simulink model "expert_random"  (R2023a)
settings: Solver=VariableStepAuto  StartTime=0.0  StopTime=1000  RelTol=1e-3
values from neighbouring files (symbols this model uses):
  A1 = 0.0154    [expert_pid_script.m]    (also in optimizer.m; parametros.m; variables.mat)
  A2 = 5e-5    (= 5e-05)    [expert_pid_script.m]    (also in optimizer.m; parametros.m; variables.mat)
  az = 1    [expert_pid_script.m]    (also in optimizer.m; parametros.m = 0.5; variables.mat = 0.5)
  g = 9.8    [expert_pid_script.m]    (also in optimizer.m; parametros.m; variables.mat)
  Q_star = ro*A2*az*sqrt(2*g*H_star)    [expert_pid_script.m]    (also in optimizer.m; parametros.m; variables.mat = 0.0616238590158)
  ro = 1000    [expert_pid_script.m]    (also in optimizer.m; parametros.m; variables.mat)
  semilla = 751    [parametros.m]    (also in variables.mat)
  st = 0.001    [parametros.m]    (also in variables.mat)
undefined symbols (not defined in the file or in its folder): DiscIntNeverNeededParam
settings Model: Creator=empg0  LastModifiedBy=empg0
settings DebuggingCC: AlgebraicLoopMsg=none

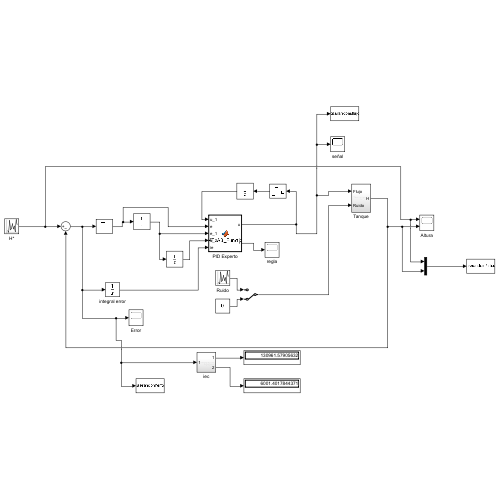
[thumbnail: Simulink's stored preview of the top-level diagram]
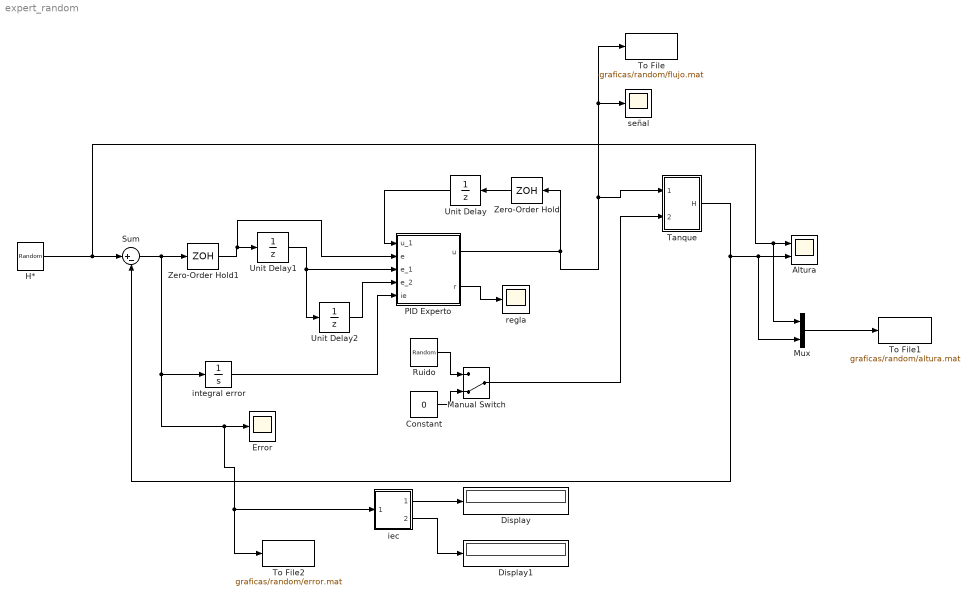
== system expert_random ==
  Altura : Scope  NumInputPorts=2
  Constant : Constant  Value=0
  Display : Display
  Display1 : Display
  Error : Scope
  H* : UniformRandomNumber  Minimum=0  Maximum=0.62  Seed=semilla  SampleTime=200
  Manual Switch : ManualSwitch  CurrentSetting=0
  Mux : Mux  Inputs=2
  PID Experto : MATLAB Function  TreatAsAtomicUnit=on
  Ruido : UniformRandomNumber  Minimum=-Q_star*0.3  Maximum=Q_star*0.3  Seed=140  SampleTime=0.5
  Sum : Sum  Inputs=|+-
  Tanque : Subsystem
  To File : ToFile  Filename=graficas/random/flujo.mat  MatrixName=flujo  SampleTime=0.25
  To File1 : ToFile  Filename=graficas/random/altura.mat  MatrixName=altura  SampleTime=0.25
  To File2 : ToFile  Filename=graficas/random/error.mat  MatrixName=error  SampleTime=0.25
  Unit Delay : UnitDelay  SampleTime=st  HasFrameUpgradeWarning=on
  Unit Delay1 : UnitDelay  SampleTime=st  HasFrameUpgradeWarning=on
  Unit Delay2 : UnitDelay  SampleTime=st  HasFrameUpgradeWarning=on
  Zero-Order Hold : ZeroOrderHold  SampleTime=st
  Zero-Order Hold1 : ZeroOrderHold  SampleTime=st
  iec : Subsystem
  integral error : Integrator
  regla : Scope
  señal : Scope
  wires:
  Tanque/1(H) -> Sum/2, Mux/2, Altura/2
  Manual Switch/1 -> Tanque/2(Ruido)
  H*/1 -> Mux/1, Altura/1, Sum/1
  Ruido/1 -> Manual Switch/1
  Constant/1 -> Manual Switch/2
  Sum/1 -> Zero-Order Hold1/1, To File2/1, iec/1(In1), Error/1, integral error/1
  Zero-Order Hold1/1 -> Unit Delay1/1, PID Experto/2(e)
  Unit Delay2/1 -> PID Experto/4(e_2)
  Unit Delay1/1 -> Unit Delay2/1, PID Experto/3(e_1)
  integral error/1 -> PID Experto/5(ie)
  PID Experto/1(u) -> To File/1, señal/1, Tanque/1(Flujo), Zero-Order Hold/1
  Zero-Order Hold/1 -> Unit Delay/1
  Unit Delay/1 -> PID Experto/1(u_1)
  PID Experto/2(r) -> regla/1
  iec/1(Out1) -> Display/1
  Mux/1 -> To File1/1
  iec/2(Out2) -> Display1/1

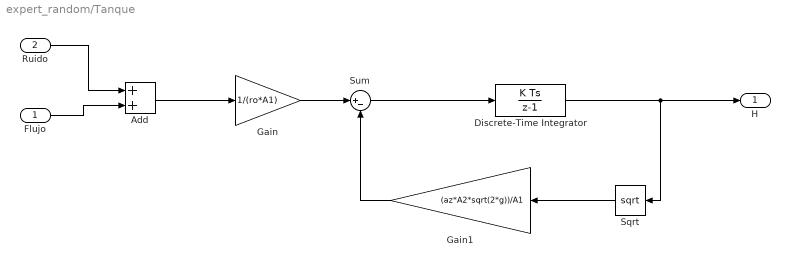
== system expert_random/Tanque ==
  Flujo : Inport
  Ruido : Inport  Port=2
  Add : Sum
  Discrete-Time Integrator : DiscreteIntegrator  SampleTime=st  LimitOutput=on  UpperSaturationLimit=0.62  LowerSaturationLimit=0  ICPrevOutput=DiscIntNeverNeededParam  ICPrevScaledInput=DiscIntNeverNeededParam
  Gain : Gain  Gain=1/(ro*A1)
  Gain1 : Gain  Gain=(az*A2*sqrt(2*g))/A1
  Sqrt : Sqrt
  Sum : Sum  Inputs=|+-
  H : Outport
  wires:
  Gain/1 -> Sum/1
  Sqrt/1 -> Gain1/1
  Gain1/1 -> Sum/2
  Add/1 -> Gain/1
  Flujo/1 -> Add/2
  Ruido/1 -> Add/1
  Sum/1 -> Discrete-Time Integrator/1
  Discrete-Time Integrator/1 -> H/1, Sqrt/1

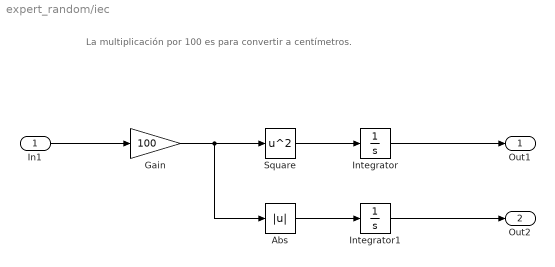
== system expert_random/iec ==
  note: La multiplicación por 100 es para convertir a centímetros.
  In1 : Inport
  Abs : Abs  SaturateOnIntegerOverflow=off
  Gain : Gain  Gain=100
  Integrator : Integrator
  Integrator1 : Integrator
  Square : Math  Operator=square  SignedPower=on  RndMeth=Zero
  Out1 : Outport
  Out2 : Outport  Port=2
  wires:
  Square/1 -> Integrator/1
  Integrator/1 -> Out1/1
  In1/1 -> Gain/1
  Gain/1 -> Abs/1, Square/1
  Integrator1/1 -> Out2/1
  Abs/1 -> Integrator1/1

== matlab function expert_random/PID Experto ==
  data: u_1 input; e input; u output; e_1 input; e_2 input; ie input; r output
function [u, r] = MATLAB_Function(u_1, e, e_1, e_2, ie)
    
    %st = load("sampling_time.mat");
    % Constantes
    H_max = 0.62;
    M1 = H_max/2;
    M2 = H_max/4;
    epsilon = 0.001; % cambié de 0.01 a 0.005
    st = 0.001; % 0.1 -> 0.001

    Qmax = 0.1; % flujo máximo
    Qmin = 0; % flujo mínimo
    
    k1 = 4.9321;
    k2 = 0.033265;
    kp = 1.06160;
    ki = 0.05; %0.03014;
    kd = -2.20023;

    de = e - e_1;
    de_1 = e_1 - e_2;
    if abs(e) > M1 % regla 1
        r = 1;
        if e > 0
            u = Qmax;
        else
            u = Qmin;
        end
    elseif abs(e) <= epsilon % regla 5
        r = 5;
        u = u_1 + kp*(e - e_1) + ki*ie;
    elseif e*de < 0 && de*de_1 < 0 % regla 4
        r = 4;
        if abs(e) >= M2
            u = u_1 + k1*kp*e;
        else
            u = u_1 + k2*kp*e;
        end
    elseif (e*de < 0 && de*de_1 > 0) || e == 0 % regla 3
        r = 3;
        u = u_1;
    elseif e*de > 0 || de == 0 % regla 2
        % funcionaba mejor cuando la regla 2 era pid normal
        r = 2;
        if abs(e) >= M2
            %control fuerte
            u = u_1 + k1*kp*(e - e_1) + k1*ki*e_1 + k1*kd*(e - 2*e_1 + e_2);
        else
            %control débil
            u = u_1 + kp*(e - e_1) + ki*e + kd*(e - 2*e_1 + e_2);
        end
    else
        r = 0;
        u = kp*e + (kd*de)/st + ki*ie;
    end
    if u > 0.1
        u = 0.1;
    end
    if u < 0
        u = 0;
    end
